simulink model "VariantSubsystemModel1"  (R2017a)
settings: Solver=FixedStepDiscrete  StartTime=0.0  StopTime=10.0  RelTol=1e-3
PreLoadFcn:
  | VSS_LINEAR_CONTROLLER=Simulink.Variant('VSS_MODE==1')
  | VSS_NONLINEAR_CONTROLLER=Simulink.Variant('VSS_MODE==2')
  | 
  | VSS_MODE=2
model workspace (MAT data in the model file):
  M_heater_air = 3600
  T_Heater = 50
  c_air = 1005.4
Description:
  | Variant Subsystems
  | 
  | This model illustrates Simulink(R) variant subsystems. Variant subsystems let
  | you provide multiple implementations to a subsystem where only one
  | implementation is active during simulation. You can programmatically swap out
  | the active implementation and replace it with one of the other implementations
  | without modifying the model.
settings Model: FPTRunName=Active  Creator=The MathWorks, Inc.  LastModifiedBy=dell
settings DataIOCC: LimitDataPoints=on  SaveFormat=Array
settings OptimizationCC: DefaultParameterBehavior=Inlined  UseDivisionForNetSlopeComputation=on  UseFloatMulNetSlope=on  InlineInvariantSignals=on  PassReuseOutputArgsAs=Individual arguments  ExpressionDepthLimit=2147483647  ZeroExternalMemoryAtStartup=off  ZeroInternalMemoryAtStartup=off  NoFixptDivByZeroProtection=on  EfficientFloat2IntCast=on  LifeSpan=1
settings DebuggingCC: UnderspecifiedInitializationDetection=Classic  MergeDetectMultiDrivingBlocksExec=none  SolverPrmCheckMsg=warning  ParameterTunabilityLossMsg=error  FcnCallInpInsideContextMsg=warning  StateNameClashWarn=warning  SFUnexpectedBacktrackingDiag=warning  SFNoUnconditionalDefaultTransitionDiag=warning  SFExecutionAtInitializationDiag=none
settings ModelReferenceCC: PropagateSignalLabelsOutOfModel=off
settings SFSimCC: MATLABDynamicMemAlloc=off
settings RTWCC: SystemTargetFile=autosar.tlc  GenCodeOnly=on  PackageGeneratedCodeAndArtifacts=on  PackageName=VariantSubsystemModel  TemplateMakefile=ert_default_tmf  Description=AUTOSAR  GenerateReport=on  IncludeHyperlinkInReport=on  LaunchReport=on  GenerateTraceInfo=on  GenerateTraceReport=on  GenerateTraceReportSl=on  GenerateTraceReportSf=on  GenerateTraceReportEml=on  GenerateCodeMetricsReport=on
settings CodeAppCC: ForceParamTrailComments=on  IgnoreCustomStorageClasses=off  OperatorAnnotations=on  SimulinkDataObjDesc=on  SFDataObjDesc=on  MATLABFcnDesc=on  CustomSymbolStrGlobalVar=rt$N$M  CustomSymbolStrType=$N$M  CustomSymbolStrFcn=$N$M$F  CustomSymbolStrMacro=$N$M  InsertBlockDesc=on  MATLABSourceComments=on
settings STFCustomTargetCC: MultiwordLength=256  ParMdlRefBuildCompliant=on  CompOptLevelCompliant=on  IncludeMdlTerminateFcn=off  CombineOutputUpdateFcns=on  CombineSignalStateStructs=on  SuppressErrorStatus=on  ERTFirstTimeCompliant=on  ERTCustomFileBanners=on  SupportAbsoluteTime=off  SupportNonFinite=off  SupportComplex=off  SupportContinuousTime=off  SupportNonInlinedSFcns=off  RemoveResetFunc=on  MATLABClassNameForMDSCustomization=Simulink.SoftwareTarget.ERTCustomization  AutosarCompliant=on  GRTInterface=off  UseToolchainInfoCompliant=on  LookupTableObjectStructAxisOrder=2,1,3,4,...  SystemTargetFile=autosar.tlc
settings ERTTargetCC: ConcurrentExecutionCompliant=off  IncludeMdlTerminateFcn=off  CombineSignalStateStructs=on  SuppressErrorStatus=on  SupportAbsoluteTime=off  SupportNonFinite=off  SupportComplex=off  ModelStepFunctionPrototypeControlCompliant=off  CPPClassGenCompliant=off  AutosarCompliant=on  LookupTableObjectStructAxisOrder=2,1,3,4,...  InlinedParameterPlacement=NonHierarchical  ERTCustomFileTemplate=example_file_process.tlc  ERTFilePackagingFormat=CompactWithDataFile
settings ConfigComp: CovMetricSettings=dw  CovHtmlReporting=on  CovSaveCumulativeToWorkspaceVar=on  CovSaveSingleToWorkspaceVar=on  CovExternalEMLEnable=off  CovSFcnEnable=off

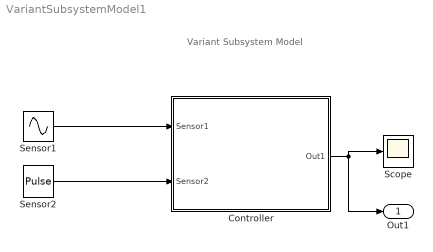
== system VariantSubsystemModel1 ==
  note: Variant Subsystem Model
  Controller : Subsystem  Variant=on
  Scope : Scope
  Sensor1 : Sin  SineType=Sample based  Amplitude=10  Bias=20  Frequency=0.5  SampleTime=1
  Sensor2 : DiscretePulseGenerator  Period=10  PulseWidth=5
  Out1 : Outport
  wires:
  Controller/1(Out1) -> Scope/1, Out1/1
  Sensor2/1 -> Controller/2(Sensor2)
  Sensor1/1 -> Controller/1(Sensor1)

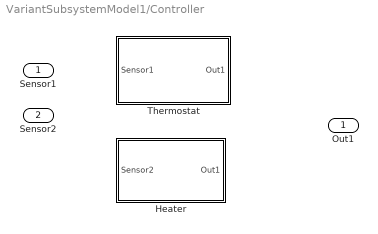
== system VariantSubsystemModel1/Controller ==
  Sensor1 : Inport
  Sensor2 : Inport  Port=2
  Heater : Subsystem  VariantControl=VSS_HEATER
  Thermostat : Subsystem  VariantControl=VSS_THERMOSTAT
  Out1 : Outport

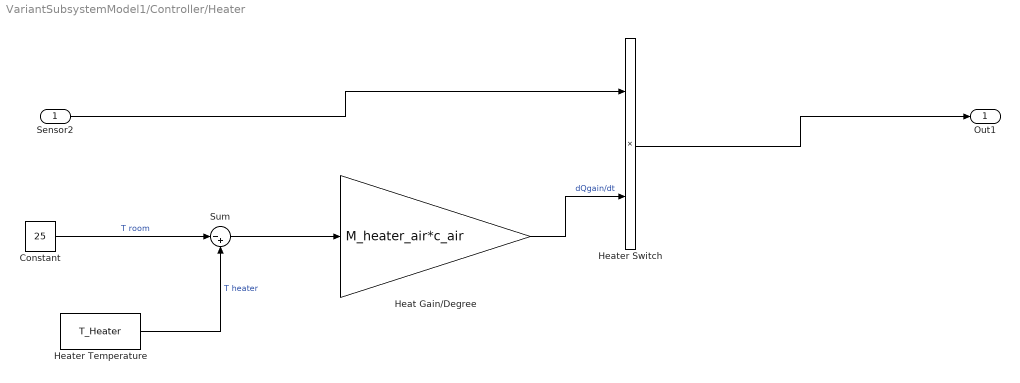
== system VariantSubsystemModel1/Controller/Heater ==
  Sensor2 : Inport
  Constant : Constant  Value=25
  Heat Gain/Degree : Gain  Gain=M_heater_air*c_air
  Heater Switch : Product
  Heater Temperature : Constant  Value=T_Heater
  Sum : Sum  Inputs=|-+
  Out1 : Outport
  wires:
  Constant/1 -> Sum/1  "T room"
  Heater Temperature/1 -> Sum/2  "T heater"
  Sum/1 -> Heat Gain/Degree/1
  Sensor2/1 -> Heater Switch/1
  Heat Gain/Degree/1 -> Heater Switch/2  "dQgain/dt"
  Heater Switch/1 -> Out1/1

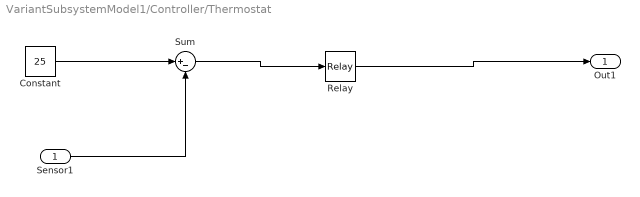
== system VariantSubsystemModel1/Controller/Thermostat ==
  "Sensor1 " : Inport
  Constant : Constant  Value=25
  Relay : Relay  OnSwitchValue=2  OffSwitchValue=-2
  Sum : Sum  Inputs=|+-
  "Out1 " : Outport
  wires:
  Constant/1 -> Sum/1
  "Sensor1 "/1 -> Sum/2
  Sum/1 -> Relay/1
  Relay/1 -> "Out1 "/1
